simulink model "IEEE5BusSystemModel_std_UFLS"  (R2019b)
settings: Solver=ode4  StartTime=0.0  StopTime=300  MaxStep=1e-4  RelTol=1e-3
InitFcn:
  | startup_RTS
values from neighbouring files (symbols this model uses):
  C = b/(2*pi*60*Zn)    [startup_RTS.m]
  C0 = C/3    [startup_RTS.m]
  fn = 50    [startup_RTS.m]
  In = Sn/(sqrt(3)*Vn)    [startup_RTS.m]
  L = x*Zn/(2*pi*60)    [startup_RTS.m]
  L0 = 3*L    [startup_RTS.m]
  len = ceil(0.95*300000*T_prop)    [startup_RTS.m]
  PL1 = 300e6    (= 300000000)    [startup_RTS.m]
  PL2 = 300e6    (= 300000000)    [startup_RTS.m]
  PL3 = 300e6    (= 300000000)    [startup_RTS.m]
  QL1 = 30e6    (= 30000000)    [startup_RTS.m]
  QL2 = 30e6    (= 30000000)    [startup_RTS.m]
  QL3 = 30e6    (= 30000000)    [startup_RTS.m]
  R = r*Zn    [startup_RTS.m]
  R0 = 3*R    [startup_RTS.m]
  Sn = 1000e6    (= 1000000000)    [startup_RTS.m]
  t_cont = 100    [startup_RTS.m]
  Vn = 345e3    (= 345000)    [startup_RTS.m]
undefined symbols (not defined in the file or in its folder): D1, Delta
libraries: powerlib x42, powerlib_meascontrol x39, dspswit3 x10, dspstat3 x3, sps_avr x3, spsExcitationSystemModel x3
(part 1 of 7)
settings Model: Creator=Rodney Tan  LastModifiedBy=zuo
settings SolverCC: AutoInsertRateTranBlk=on
settings DataIOCC: ReturnWorkspaceOutputs=off
settings OptimizationCC: LifeSpan=inf
settings DebuggingCC: UnconnectedInputMsg=none  UnconnectedOutputMsg=none  UnconnectedLineMsg=none  SFUnexpectedBacktrackingDiag=warning  SFNoUnconditionalDefaultTransitionDiag=warning  SFExecutionAtInitializationDiag=none  ArithmeticOperatorsInVariantConditions=warning
settings SFSimCC: SimUseLocalCustomCode=off  CustomCodeUndefinedFunction=UseInterfaceOnly
settings RTWCC: RTWUseLocalCustomCode=off
settings CodeAppCC: StateflowObjectComments=on
settings GRTTargetCC: TargetLangStandard=C89/C90 (ANSI)  GeneratePreprocessorConditionals=Disable all
settings ConfigComp: CovMetricSettings=dw  CovHtmlReporting=on  CovSaveCumulativeToWorkspaceVar=on  CovSaveSingleToWorkspaceVar=on  CovExternalEMLEnable=off
settings SimscapeCC: SimscapeNormalizeSystem=off

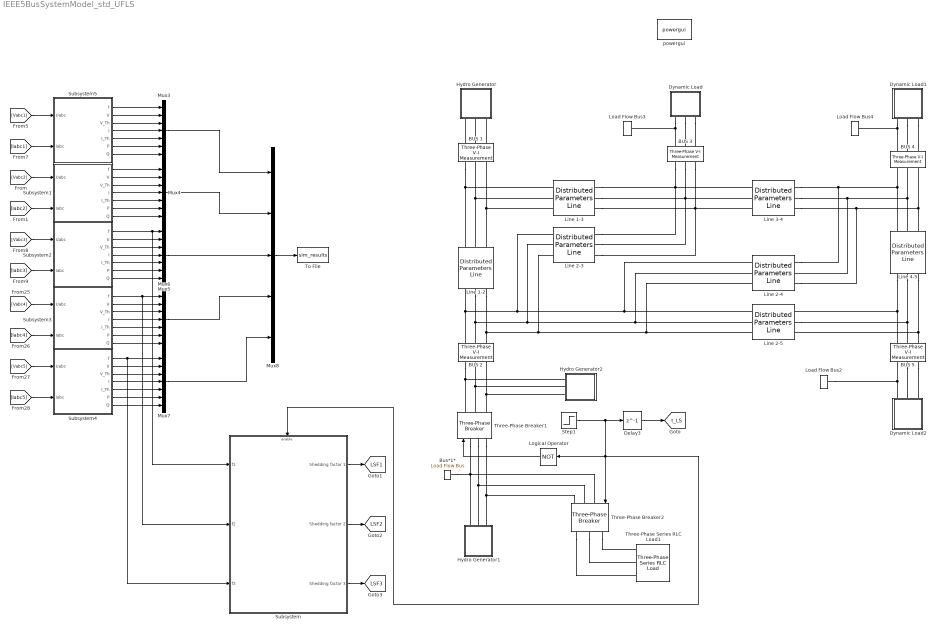
== system IEEE5BusSystemModel_std_UFLS ==
  BUS 1 : powerlib/Measurements/Three-Phase V-I Measurement  VoltageMeasurement=phase-to-ground  SetLabelV=on  LabelV=Vabc1  Vpu=off  VpuLL=off  CurrentMeasurement=yes  SetLabelI=on  LabelI=Iabc1  Ipu=off  Pbase=100e6  Vbase=500e3  OutputType=Complex  PhasorSimulation=off  PSBequivalent=0
      settings: SourceProductName=Simscape Electrical
  BUS 2 : powerlib/Measurements/Three-Phase V-I Measurement  VoltageMeasurement=phase-to-ground  SetLabelV=on  LabelV=Vabc2  Vpu=off  VpuLL=off  CurrentMeasurement=yes  SetLabelI=on  LabelI=Iabc2  Ipu=off  Pbase=100e6  Vbase=500e3  OutputType=Complex  PhasorSimulation=off  PSBequivalent=0
      settings: SourceProductName=Simscape Electrical
  BUS 3 : powerlib/Measurements/Three-Phase V-I Measurement  VoltageMeasurement=phase-to-ground  SetLabelV=on  LabelV=Vabc3  Vpu=off  VpuLL=off  CurrentMeasurement=yes  SetLabelI=on  LabelI=Iabc3  Ipu=off  Pbase=100e6  Vbase=500e3  OutputType=Complex  PhasorSimulation=off  PSBequivalent=0
      settings: SourceProductName=Simscape Electrical
  BUS 4 : powerlib/Measurements/Three-Phase V-I Measurement  VoltageMeasurement=phase-to-ground  SetLabelV=on  LabelV=Vabc4  Vpu=off  VpuLL=off  CurrentMeasurement=yes  SetLabelI=on  LabelI=Iabc4  Ipu=off  Pbase=100e6  Vbase=500e3  OutputType=Complex  PhasorSimulation=off  PSBequivalent=0
      settings: SourceProductName=Simscape Electrical
  BUS 5 : powerlib/Measurements/Three-Phase V-I Measurement  VoltageMeasurement=phase-to-ground  SetLabelV=on  LabelV=Vabc5  Vpu=off  VpuLL=off  CurrentMeasurement=yes  SetLabelI=on  LabelI=Iabc5  Ipu=off  Pbase=100e6  Vbase=500e3  OutputType=Complex  PhasorSimulation=off  PSBequivalent=0
      settings: SourceProductName=Simscape Electrical
  Bus*1* : powerlib/Measurements/Load Flow Bus  LConnTagsString=a  Phases=single  Connectors=on one side  ID=BUS_2_2  Vbase=345e3  Vref=1  Vangle=0  VLF=1.079  VLFb=1  VLFc=1  angleLF=22.73  angleLFb=0  angleLFc=0
      settings: SourceProductName=Simscape Electrical
  Delay3 : Delay  DelayLength=1  InitialCondition=0
  Dynamic Load : Subsystem
  Dynamic Load1 : Subsystem
  Dynamic Load2 : Subsystem
  Hydro Generator : Subsystem  mask{pTotal=1000, fNom=50, vNom=22}
      mask prompts: pTotal "Total generation (MWatt)"; fNom "Nominal frequency (Hz)"; vNom "Nominal L-L voltage (kV)"
      mask DialogControl ParameterGroupVar Prompt: HSG paramters
  Hydro Generator1 : Subsystem  mask{pTotal=1000, fNom=50, vNom=22}
      mask prompts: pTotal "Total generation (MWatt)"; fNom "Nominal frequency (Hz)"; vNom "Nominal L-L voltage (kV)"
      mask DialogControl ParameterGroupVar Prompt: HSG paramters
  Hydro Generator2 : Subsystem  mask{pTotal=1000, fNom=50, vNom=22}
      mask prompts: pTotal "Total generation (MWatt)"; fNom "Nominal frequency (Hz)"; vNom "Nominal L-L voltage (kV)"
      mask DialogControl ParameterGroupVar Prompt: HSG paramters
  Line 1-2 : powerlib/Elements/Distributed Parameters Line  Phases=3  Frequency=50  Resistance=[R(1) R0(1)]/len(1)  Inductance=[L(1) L0(1)]/len(1)  Capacitance=[C(1) C0(1)]/len(1)  Length=len(1)  x1=[-0.000175 -6.89085295701592e-11 283434.108559995 -241348.137066872;-0.00015 -2.16346671578411e-11 285320.892161224 -239114.627668055;-0.000125 2.56405297826555e-11 287190.075825844 -236866.368552673;-0.0001 7.29141450944975e-11 289041.544253801 -234603.498403938;-7.5e-05 1.20183262718414e-10 290875.183237801 -232326.156806341;-5e-05 1.67444966872572e-10 292690.879670354 -230034.484237038;-2.5e-05 2.14696342232437e-10 294488.521550753 -227728.622057188]  x2=[-0.000175 1.27432514229788e-09 287186.952133436 -239007.168100233;-0.00015 1.33160990762763e-09 289055.234274348 -236744.256496373;-0.000125 1.38881253298583e-09 290905.686126838 -234466.741391606;-0.0001 1.44592948984511e-09 292738.19354632 -232174.763273793;-7.5e-05 1.50295725496252e-09 294552.643495105 -229868.463522941;-5e-05 1.55989231059688e-09 296348.924049371 -227547.984402482;-2.5e-05 1.61673114472578e-09 298126.924406074 -225213.469050498]  x3=[-0.000175 -3.16049108701691e-11 2846.8299317029 -2460.69390485512;-0.00015 -3.08579762390022e-11 2866.06819220975 -2438.25927190657;-0.000125 -3.01091381425069e-11 2885.12966013012 -2415.6742356409;-0.0001 -2.93584427725443e-11 2904.01315966288 -2392.94018920953;-7.5e-05 -2.86059364355409e-11 2922.71752598482 -2370.05853495554;-5e-05 -2.78516655496321e-11 2941.24160532254 -2347.03068432714;-2.5e-05 -2.70956766417991e-11 2959.58425502355 -2323.85805779063]  x4=[-0.000175 3.74399132665437e-11 1776.05546983702 -1633.69511882766;-0.00015 3.68414015455268e-11 1788.83157054831 -1619.69575008179;-0.000125 3.6240617273324e-11 1801.49732770218 -1605.59647087261;-0.0001 3.56375975091392e-11 1814.05196001507 -1591.39815091007;-7.5e-05 3.5032379450072e-11 1826.49469305811 -1577.10166601343;-5e-05 3.44250004288231e-11 1838.82475930493 -1562.70789805721;-2.5e-05 3.38154979113915e-11 1851.04139817896 -1548.21773491684]  x5=0.000159154943091895  V1=ones(3,3)  V2=ones(3,3)  I1=ones(3,3)  I2=ones(3,3)  nHarmo=1  Measurements=None
      settings: SourceProductName=Simscape Electrical
  Line 1-3 : powerlib/Elements/Distributed Parameters Line  Phases=3  Frequency=50  Resistance=[R(2) R0(2)]/len(2)  Inductance=[L(2) L0(2)]/len(2)  Capacitance=[C(2) C0(2)]/len(2)  Length=len(2)  x1=[-0.0003 9.72648087730306e-10 277582.158753036 -250097.820068359;-0.000275 1.03025169047578e-09 279537.841922512 -247910.001458296;-0.00025 1.08779174244406e-09 281476.281881158 -245706.890591581;-0.000225 1.14526469429371e-09 283397.359056865 -243488.623366473;-0.0002 1.20266700082234e-09 285300.954948545 -241255.336616141;-0.000175 1.25999512118529e-09 287186.952133436 -239007.168100233;-0.00015 1.31724551911407e-09 289055.234274348 -236744.256496373;-0.000125 1.37441466313444e-09 290905.686126838 -234466.741391606;-0.0001 1.43149902678431e-09 292738.19354632 -232174.763273793;-7.5e-05 1.48849508883126e-09 294552.643495105 -229868.463522941;-5e-05 1.54539933348968e-09 296348.924049371 -227547.984402482;-2.5e-05 1.60220825063774e-09 298126.924406074 -225213.469050498]  x2=[-0.0003 1.7615419409433e-09 265030.630049931 -256880.545118797;-0.000275 1.80458215738261e-09 267039.971168693 -254791.095722945;-0.00025 1.84751105869411e-09 269032.840004163 -252685.929612136;-0.000225 1.89032599682095e-09 271009.113626804 -250565.176642931;-0.0002 1.93302433073608e-09 272968.670130749 -248428.967633363;-0.000175 1.97560342660514e-09 274911.388641323 -246277.434354866;-0.00015 2.01806065794892e-09 276837.149322498 -244110.709524149;-0.000125 2.0603934058054e-09 278745.833384283 -241928.926795004;-0.0001 2.10259905889129e-09 280637.323090054 -239732.220750067;-7.5e-05 2.1446750137631e-09 282511.501763818 -237520.726892514;-5e-05 2.18661867497775e-09 284368.253797405 -235294.581637705;-2.5e-05 2.22842745525262e-09 286207.464657603 -233053.922304763]  x3=[-0.0003 2.71909208464363e-11 572.658083588603 -630.300021251127;-0.000275 2.72692719095188e-11 577.590736411029 -625.782972903441;-0.00025 2.73459408754602e-11 582.487760716138 -621.227323314286;-0.000225 2.74209230149575e-11 587.348854432404 -616.633353497587;-0.0002 2.74942137027591e-11 592.173717704668 -612.001346831042;-0.000175 2.75658084179503e-11 596.962052912636 -607.33158903864;-0.00015 2.76357027442317e-11 601.713564689239 -602.624368173039;-0.000125 2.7703892370192e-11 606.427959938848 -597.879974597795;-0.0001 2.7770373089574e-11 611.104947855357 -593.098700969452;-7.5e-05 2.78351408015336e-11 615.744239940121 -588.280842219489;-5e-05 2.78981915108934e-11 620.345550019751 -583.426695536128;-2.5e-05 2.79595213283886e-11 624.908594263768 -578.536560346]  x4=[-0.0003 -2.32249180429763e-11 1364.78490116338 -1354.69627143181;-0.000275 -2.31577834751214e-11 1375.38246353659 -1343.93559538929;-0.00025 -2.30892204260988e-11 1385.89518584082 -1333.09201906874;-0.000225 -2.30192331252005e-11 1396.32241960183 -1322.16621135304;-0.0002 -2.29478258895727e-11 1406.66352161874 -1311.15884619745;-0.000175 -2.28750031239501e-11 1416.91785400366 -1300.07060258813;-0.00015 -2.2800769320384e-11 1427.08478422106 -1288.90216450015;-0.000125 -2.27251290579649e-11 1437.16368512681 -1277.6542208554;-0.0001 -2.26480870025407e-11 1447.15393500681 -1266.32746548002;-7.5e-05 -2.25696479064281e-11 1457.05491761539 -1254.92259706163;-5e-05 -2.24898166081201e-11 1466.86602221332 -1243.44031910624;-2.5e-05 -2.24085980319872e-11 1476.58664360543 -1231.88133989485]  x5=0.000290575841566274  V1=ones(3,3)  V2=ones(3,3)  I1=ones(3,3)  I2=ones(3,3)  nHarmo=1  Measurements=None
      settings: SourceProductName=Simscape Electrical
  Line 2-3 : powerlib/Elements/Distributed Parameters Line  Phases=3  Frequency=50  Resistance=[R(3) R0(3)]/len(3)  Inductance=[L(3) L0(3)]/len(3)  Capacitance=[C(3) C0(3)]/len(3)  Length=len(3)  x1=[-0.00025 -7.55210722613573e-10 277669.32737874 -247958.793830222;-0.000225 -7.06042606866762e-10 279608.208168973 -245770.356539619;-0.0002 -6.56830939086201e-10 281529.841407855 -243566.758975743;-0.000175 -6.07578754879368e-10 283434.108559994 -241348.137066872;-0.00015 -5.58289092352982e-10 285320.892161224 -239114.627668055;-0.000125 -5.08964991925604e-10 287190.075825844 -236866.368552673;-0.0001 -4.59609496140084e-10 289041.5442538 -234603.498403938;-7.5e-05 -4.10225649475888e-10 290875.1832378 -232326.156806341;-5e-05 -3.60816498161298e-10 292690.879670354 -230034.484237038;-2.5e-05 -3.11385089985503e-10 294488.521550752 -227728.622057188]  x2=[-0.00025 1.84751105869411e-09 269032.840004163 -252685.929612136;-0.000225 1.89032599682095e-09 271009.113626804 -250565.176642931;-0.0002 1.93302433073608e-09 272968.670130749 -248428.967633363;-0.000175 1.97560342660514e-09 274911.388641323 -246277.434354866;-0.00015 2.01806065794892e-09 276837.149322498 -244110.709524149;-0.000125 2.0603934058054e-09 278745.833384283 -241928.926795004;-0.0001 2.10259905889129e-09 280637.323090054 -239732.220750067;-7.5e-05 2.1446750137631e-09 282511.501763818 -237520.726892514;-5e-05 2.18661867497775e-09 284368.253797405 -235294.581637705;-2.5e-05 2.22842745525262e-09 286207.464657603 -233053.922304763]  x3=[-0.00025 2.75995009114326e-11 652.704108135299 -678.234675376389;-0.000225 2.79468601247303e-11 658.010768792704 -673.087474371481;-0.0002 2.82924954440539e-11 663.276840246383 -667.898754160629;-0.000175 2.8636385548989e-11 668.501997660243 -662.668834808537;-0.00015 2.8978509226774e-11 673.685918721962 -657.398038921264;-0.000125 2.9318845373609e-11 678.828283662869 -652.08669162633;-0.0001 2.96573729959572e-11 683.928775277674 -646.735120552653;-7.5e-05 2.99940712118403e-11 688.987078944027 -641.343655810347;-5e-05 3.03289192521264e-11 694.002882641933 -635.912629970351;-2.5e-05 3.0661896461811e-11 698.975876972991 -630.442378043924]  x4=[-0.00025 -2.89166148510431e-11 1397.97485671835 -1338.51479489178;-0.000225 -2.91605454608319e-11 1408.44430570704 -1327.49394730035;-0.0002 -2.94026773108183e-11 1418.82687521659 -1316.39121362919;-0.000175 -2.96429954651693e-11 1429.12192480121 -1305.20727874722;-0.00015 -2.98814850999289e-11 1439.32881941374 -1293.94283253223;-0.000125 -3.01181315039332e-11 1449.44692944484 -1282.5985698283;-0.0001 -3.03529200797173e-11 1459.47563076183 -1271.17519040301;-7.5e-05 -3.05858363444158e-11 1469.41430474717 -1259.67339890421;-5e-05 -3.08168659306565e-11 1479.26233833664 -1248.09390481657;-2.5e-05 -3.10459945874462e-11 1489.01912405713 -1236.43742241784]  x5=0.000225079079039277  V1=ones(3,3)  V2=ones(3,3)  I1=ones(3,3)  I2=ones(3,3)  nHarmo=1  Measurements=None
      settings: SourceProductName=Simscape Electrical
  Line 2-4 : powerlib/Elements/Distributed Parameters Line  Phases=3  Frequency=50  Resistance=[R(4) R0(4)]/len(4)  Inductance=[L(4) L0(4)]/len(4)  Capacitance=[C(4) C0(4)]/len(4)  Length=len(4)  x1=[-0.00025 -7.55210722613573e-10 277669.32737874 -247958.793830222;-0.000225 -7.06042606866762e-10 279608.208168973 -245770.356539619;-0.0002 -6.56830939086201e-10 281529.841407855 -243566.758975743;-0.000175 -6.07578754879368e-10 283434.108559994 -241348.137066872;-0.00015 -5.58289092352982e-10 285320.892161224 -239114.627668055;-0.000125 -5.08964991925604e-10 287190.075825844 -236866.368552673;-0.0001 -4.59609496140084e-10 289041.5442538 -234603.498403938;-7.5e-05 -4.10225649475888e-10 290875.1832378 -232326.156806341;-5e-05 -3.60816498161298e-10 292690.879670354 -230034.484237038;-2.5e-05 -3.11385089985503e-10 294488.521550752 -227728.622057188]  x2=[-0.00025 1.04438515929711e-09 268312.349842603 -253068.826139404;-0.000225 1.09016772438184e-09 270291.652916932 -250953.720015734;-0.0002 1.13588304278619e-09 272254.283128921 -248823.133884516;-0.000175 1.18152829457397e-09 274200.119414295 -246677.199170339;-0.00015 1.22710066413105e-09 276129.041744706 -244516.048244564;-0.000125 1.272597340339e-09 278040.931135137 -242339.814417159;-0.0001 1.31801551674853e-09 279935.669651247 -240148.631928479;-7.5e-05 1.36335239175258e-09 281813.140416638 -237942.63594098;-5e-05 1.40860516875915e-09 283673.227620069 -235721.962530887;-2.5e-05 1.45377105636378e-09 285515.816522601 -233486.748679795]  x3=[-0.00025 1.8608938054906e-11 620.73944245554 -651.189706585723;-0.000225 1.88719827024415e-11 625.834680289495 -646.294387025691;-0.0002 1.91338632371889e-11 630.891313692424 -641.359200983548;-0.000175 1.93945635051234e-11 635.909030747361 -636.384452884818;-0.00015 1.96540674250242e-11 640.887521937884 -631.370449595395;-0.000125 1.99123589894674e-11 645.826480167203 -626.31750040262;-0.0001 2.01694222658125e-11 650.725600777111 -621.225916996202;-7.5e-05 2.04252413971858e-11 655.584581566771 -616.096013448989;-5e-05 2.06798006034582e-11 660.403122811362 -610.928106197594;-2.5e-05 2.09330841822189e-11 665.180927280561 -605.722514022881]  x4=[-0.00025 -1.78719646829918e-11 1427.09295112561 -1366.9449250186;-0.000225 -1.80290498138173e-11 1437.78478964706 -1355.69450993648;-0.0002 -1.8185022827926e-11 1448.38793883011 -1344.36046923109;-0.000175 -1.83398741041675e-11 1458.90174462257 -1332.94350203946;-0.00015 -1.84935940905857e-11 1469.32555848339 -1321.44431261389;-0.000125 -1.86461733050078e-11 1479.65873742262 -1309.86361027857;-0.0001 -1.87976023356291e-11 1489.90064404111 -1298.20210938575;-7.5e-05 -1.89478718415938e-11 1500.05064656981 -1286.46052927175;-5e-05 -1.90969725535708e-11 1510.10811890877 -1274.63959421254;-2.5e-05 -1.9244895274326e-11 1520.07244066571 -1262.74003337907]  x5=0.000225079079039277  V1=ones(3,3)  V2=ones(3,3)  I1=ones(3,3)  I2=ones(3,3)  nHarmo=1  Measurements=None
      settings: SourceProductName=Simscape Electrical
  Line 2-5 : powerlib/Elements/Distributed Parameters Line  Phases=3  Frequency=50  Resistance=[R(5) R0(5)]/len(5)  Inductance=[L(5) L0(5)]/len(5)  Capacitance=[C(5) C0(5)]/len(5)  Length=len(5)  x1=[-0.000175 -6.07578754879368e-10 283434.108559994 -241348.137066872;-0.00015 -5.58289092352982e-10 285320.892161224 -239114.627668055;-0.000125 -5.08964991925604e-10 287190.075825844 -236866.368552673;-0.0001 -4.59609496140084e-10 289041.5442538 -234603.498403938;-7.5e-05 -4.10225649475888e-10 290875.1832378 -232326.156806341;-5e-05 -3.60816498161298e-10 292690.879670354 -230034.484237038;-2.5e-05 -3.11385089985503e-10 294488.521550752 -227728.622057188]  x2=[-0.000175 -1.8455816791541e-10 274204.431996219 -246369.649771894;-0.00015 -1.4365476424163e-10 276130.938727661 -244208.474456257;-0.000125 -1.02742499265318e-10 278040.412402109 -242032.23521159;-0.0001 -6.18238966476901e-11 279932.735234233 -239841.066278583;-7.5e-05 -2.09014804409006e-11 281807.790496646 -237635.102818854;-5e-05 2.00222250676572e-11 283665.462527109 -235414.480906623;-2.5e-05 6.09446955110597e-11 285505.636735659 -233179.337520308]  x3=[-0.000175 3.21776861319045e-11 522.866429808054 -510.097497337829;-0.00015 3.22539034337297e-11 526.856562179851 -505.975213824819;-0.000125 3.23281311628617e-11 530.814195557177 -501.821719377265;-0.0001 3.24003647405844e-11 534.739085814563 -497.637270202268;-7.5e-05 3.24705997111906e-11 538.63099084629 -493.422124416364;-5e-05 3.25388317422565e-11 542.489670581323 -489.176542029601;-2.5e-05 3.26050566249089e-11 546.31488699812 -484.900784929497]  x4=[-0.000175 -3.21081774868052e-11 1734.08510457111 -1566.21499511989;-0.00015 -3.20776836134101e-11 1746.33252307936 -1552.54734768471;-0.000125 -3.20452110373903e-11 1758.47221957162 -1538.78393181597;-0.0001 -3.20107617618073e-11 1770.50344521424 -1524.92559650599;-7.5e-05 -3.19743379116547e-11 1782.42545786453 -1510.97319660219;-5e-05 -3.19359417337271e-11 1794.23752211662 -1496.92759275429;-2.5e-05 -3.18955755964816e-11 1805.93890934672 -1482.78965136132]  x5=0.000159154943091895  V1=ones(3,3)  V2=ones(3,3)  I1=ones(3,3)  I2=ones(3,3)  nHarmo=1  Measurements=None
      settings: SourceProductName=Simscape Electrical
  Line 3-4 : powerlib/Elements/Distributed Parameters Line  Phases=3  Frequency=50  Resistance=[R(6) R0(6)]/len(6)  Inductance=[L(6) L0(6)]/len(6)  Capacitance=[C(6) C0(6)]/len(6)  Length=len(6)  x1=[-7.5e-05 2.14450359391277e-09 282511.501763818 -237520.726892514;-5e-05 2.18650438920275e-09 284368.253797405 -235294.581637705;-2.5e-05 2.22837031060265e-09 286207.464657603 -233053.922304763]  x2=[-7.5e-05 1.36335239175258e-09 281813.140416638 -237942.63594098;-5e-05 1.40860516875915e-09 283673.227620069 -235721.962530887;-2.5e-05 1.45377105636378e-09 285515.816522601 -233486.748679795]  x3=[-7.5e-05 -6.39975385908229e-11 1707.26151893148 -1486.29546105194;-5e-05 -6.42947165516981e-11 1718.8820864755 -1472.84094214289;-2.5e-05 -6.45879285116012e-11 1730.39662527578 -1459.29557146682]  x4=[-7.5e-05 5.80762461840834e-11 2107.15394566836 -1794.76808776156;-5e-05 5.87994680738186e-11 2121.18489524858 -1778.16333946726;-2.5e-05 5.95190629353929e-11 2135.08500015278 -1761.44890568229]  x5=6.49747334361397e-05  V1=ones(3,3)  V2=ones(3,3)  I1=ones(3,3)  I2=ones(3,3)  nHarmo=1  Measurements=None
      settings: SourceProductName=Simscape Electrical
  Line 4-5 : powerlib/Elements/Distributed Parameters Line  Phases=3  Frequency=50  Resistance=[R(7) R0(7)]/len(7)  Inductance=[L(7) L0(7)]/len(7)  Capacitance=[C(7) C0(7)]/len(7)  Length=len(7)  x1=[-0.0003 -4.02656590795237e-10 264320.598105925 -256944.934494444;-0.000275 -3.61902544883196e-10 266330.466826514 -254861.059625176;-0.00025 -3.21126175117472e-10 268323.907029381 -252761.463725248;-0.000225 -2.80329996776628e-10 270300.795749744 -250646.276307624;-0.0002 -2.39516526361111e-10 272261.011043794 -248515.627847028;-0.000175 -1.98688281438024e-10 274204.431996219 -246369.649771894;-0.00015 -1.57847780485833e-10 276130.938727661 -244208.474456257;-0.000125 -1.16997542739012e-10 278040.412402109 -242032.23521159;-0.0001 -7.6140088032647e-11 279932.735234233 -239841.066278583;-7.5e-05 -3.52779366470004e-11 281807.790496646 -237635.102818854;-5e-05 5.58639084795246e-12 283665.462527109 -235414.480906623;-2.5e-05 4.64503737480036e-11 285505.636735659 -233179.337520308]  x2=[-0.0003 9.5262958939744e-10 264304.214498806 -257252.077448191;-0.000275 9.98538171616254e-10 266316.495998673 -255168.321785816;-0.00025 1.04438515929711e-09 268312.349842603 -253068.826139404;-0.000225 1.09016772438184e-09 270291.652916932 -250953.720015734;-0.0002 1.13588304278619e-09 272254.283128921 -248823.133884516;-0.000175 1.18152829457397e-09 274200.119414295 -246677.199170339;-0.00015 1.22710066413105e-09 276129.041744706 -244516.048244564;-0.000125 1.272597340339e-09 278040.931135137 -242339.814417159;-0.0001 1.31801551674853e-09 279935.669651247 -240148.631928479;-7.5e-05 1.36335239175258e-09 281813.140416638 -237942.63594098;-5e-05 1.40860516875915e-09 283673.227620069 -235721.962530887;-2.5e-05 1.45377105636378e-09 285515.816522601 -233486.748679795]  x3=[-0.0003 -2.58292308145759e-12 930.888255854728 -1007.97476830205;-0.000275 -2.38221400636998e-12 938.776082330799 -1000.63256707165;-0.00025 -2.18135798510122e-12 946.606000676083 -993.228642111112;-0.000225 -1.98036740739683e-12 954.377527904332 -985.763450129404;-0.0002 -1.77925467130239e-12 962.09018463114 -978.237451614732;-0.000175 -1.57803218239878e-12 969.743495103511 -970.651110806135;-0.00015 -1.37671235303697e-12 977.336987229204 -963.004895664848;-0.000125 -1.17530760157233e-12 984.870192605857 -955.299277845438;-0.0001 -9.73830351598629e-13 992.342646549877 -947.53473266671;-7.5e-05 -7.72293031181692e-13 999.753888125107 -939.711739082384;-5e-05 -5.70708072092767e-13 1007.10346017126 -931.830779651553;-2.5e-05 -3.6908790904168e-13 1014.3909093321 -923.892340508919]  x4=[-0.0003 2.44800646108232e-12 953.120272984546 -1001.55052875308;-0.000275 2.36564734954155e-12 960.956958009434 -994.033917746149;-0.00025 2.28314231372906e-12 968.73436668264 -986.455990044854;-0.000225 2.2004964429441e-12 976.452019256962 -978.817213091471;-0.0002 2.11771483517327e-12 984.109439671238 -971.118058081744;-0.000175 2.03480259677608e-12 991.706155579704 -963.35899993582;-0.00015 1.95176484216995e-12 999.241698381142 -955.540517268954;-0.000125 1.86860669351472e-12 1006.71560324778 -947.663092361985;-0.0001 1.78533328039671e-12 1014.12740915395 -939.727211131587;-7.5e-05 1.7019497395123e-12 1021.47665890455 -931.733363100297;-5e-05 1.61846121435105e-12 1028.76289916325 -923.682041366314;-2.5e-05 1.53487285487847e-12 1035.98568048043 -915.573742573089]  x5=0.000290575841566274  V1=ones(3,3)  V2=ones(3,3)  I1=ones(3,3)  I2=ones(3,3)  nHarmo=1  Measurements=None
      settings: SourceProductName=Simscape Electrical
  Load Flow Bus2 : powerlib/Measurements/Load Flow Bus  LConnTagsString=a  Phases=single  Connectors=on one side  ID=BUS_5  Vbase=345e3  Vref=1  Vangle=0  VLF=1.068  VLFb=1  VLFc=1  angleLF=21.21  angleLFb=0  angleLFc=0
      settings: SourceProductName=Simscape Electrical
  Load Flow Bus3 : powerlib/Measurements/Load Flow Bus  LConnTagsString=a  Phases=single  Connectors=on one side  ID=BUS_3  Vbase=345e3  Vref=1  Vangle=0  VLF=1.07  VLFb=1  VLFc=1  angleLF=21.29  angleLFb=0  angleLFc=0
      settings: SourceProductName=Simscape Electrical
  Load Flow Bus4 : powerlib/Measurements/Load Flow Bus  LConnTagsString=a  Phases=single  Connectors=on one side  ID=BUS_4  Vbase=345e3  Vref=1  Vangle=0  VLF=1.069  VLFb=1  VLFc=1  angleLF=21.17  angleLFb=0  angleLFc=0
      settings: SourceProductName=Simscape Electrical
  Logical Operator : Logic  Operator=NOT  AllPortsSameDT=off  OutDataTypeStr=boolean
  Mux{3..7} (5 alike) : Mux  Inputs=7
  Mux8 : Mux  Inputs=5
  Step1 : Step  Time=t_cont  SampleTime=0
  Subsystem : Subsystem
  Subsystem1 : Subsystem
  Subsystem2 : Subsystem
  Subsystem3 : Subsystem
  Subsystem4 : Subsystem
  Subsystem5 : Subsystem
  Three-Phase Series RLC Load1 : powerlib/Elements/Three-Phase Series RLC Load  LConnTagsString=A|B|C  Configuration=Y (grounded)  NominalVoltage=(345000)*1.02511  Vabc=[1e3 1e3 1e3]  Vabcp=[1e3 1e3 1e3]  NominalFrequency=50  UnbalancedPower=off  ActivePower=300e6  InductivePower=30e6  CapacitivePower=0  Pabc=[10e3 9e3 11e3]  QLabc=[100 90 110]  QCabc=[100 90 110]  Pabcp=[10e3 9e3 11e3]  QLabcp=[100 90 110]  QCabcp=[100 90 110]  Measurements=None  LoadType=constant PQ
      settings: SourceProductName=Simscape Electrical
  Three-Phase Breaker1 : powerlib/Elements/Three-Phase Breaker  InitialState=closed  SwitchA=on  SwitchB=on  SwitchC=on  SwitchTimes=[]  External=on  BreakerResistance=0.01  SnubberResistance=1e9  SnubberCapacitance=inf  Measurements=None
      settings: SourceProductName=Simscape Electrical
  Three-Phase Breaker2 : powerlib/Elements/Three-Phase Breaker  InitialState=open  SwitchA=on  SwitchB=on  SwitchC=on  SwitchTimes=[]  External=on  BreakerResistance=0.01  SnubberResistance=1e9  SnubberCapacitance=inf  Measurements=None
      settings: SourceProductName=Simscape Electrical
  To File : ToFile  Filename=sim_results  MatrixName=sim1
  powergui : powerlib/powergui  Priority=1  SimulationMode=Discrete  SampleTime=25e-6  frequency=60  Iterations=50  frequencyindice=50  Pbase=1000e6  ErrMax=0.0001  UnitsV=kV  UnitsW=MW  buscounter=3  FunctionMessages=off  echomessages=off  EnableUseOfTLC=off  CurrentSourceSwitches=off  DisableSnubberDevices=off  DisableRonSwitches=off  DisableVfSwitches=off  DisplayEquations=off  AutomaticDiscreteSolvers=off  SolverType=Tustin/Backward Euler (TBE)  Interpol=off  ExternalGateDelay=off  methode=off  Ts=100  x0status=blocks  SPID=on  SwTol=0  HookPort=off  NonlinearTolerance=1e-4  nMaxIteration=100  ContinueOnMaxIteration=off  RestoreLinks=warning  ResistiveCurrentMeasurement=off  Frange=[0:2:500]  Ylog=off  Xlog=on  ShowGrid=off  save=off  variable=ZData  structure=0  ZoomFFT=off  StartTime=0.0  cycles=1  DisplayStyle=1  fundamental=60  FreqAxis=off  MaxFrequency=1000  frequencyindicesteady=1  RmsSteady=1  display=off
      settings: SourceProductName=Simscape Electrical
  tag scope: LSF1=global, LSF2=global, LSF3=global, t_LS=global
  wires:
  Logical Operator/1 -> Three-Phase Breaker1/1
  Step1/1 -> Logical Operator/1, Subsystem/Enable, Three-Phase Breaker2/1, Delay3/1
  [Vabc1] -> Subsystem5/1(Uabc)
  [Vabc3] -> Subsystem2/1(Uabc)
  [Iabc2] -> Subsystem1/2(Iabc)
  [Iabc3] -> Subsystem2/2(Iabc)
  [Iabc1] -> Subsystem5/2(Iabc)
  [Vabc2] -> Subsystem1/1(Uabc)
  [Vabc4] -> Subsystem3/1(Uabc)
  [Iabc5] -> Subsystem4/2(Iabc)
  [Iabc4] -> Subsystem3/2(Iabc)
  [Vabc5] -> Subsystem4/1(Uabc)
  Subsystem5/1(f) -> Mux3/1
  Subsystem5/2(V) -> Mux3/2
  Subsystem5/3(V_Th) -> Mux3/3
  Subsystem5/4(I) -> Mux3/4
  Subsystem5/5(I_Th) -> Mux3/5
  Subsystem5/6(P) -> Mux3/6
  Subsystem5/7(Q) -> Mux3/7
  Subsystem1/7(Q) -> Mux4/7
  Subsystem1/6(P) -> Mux4/6
  Subsystem1/5(I_Th) -> Mux4/5
  Subsystem1/4(I) -> Mux4/4
  Subsystem1/3(V_Th) -> Mux4/3
  Subsystem1/2(V) -> Mux4/2
  Subsystem1/1(f) -> Mux4/1
  Subsystem2/1(f) -> Subsystem/1(f1), Mux5/1
  Subsystem2/2(V) -> Mux5/2
  Subsystem2/3(V_Th) -> Mux5/3
  Subsystem2/4(I) -> Mux5/4
  Subsystem2/5(I_Th) -> Mux5/5
  Subsystem2/6(P) -> Mux5/6
  Subsystem2/7(Q) -> Mux5/7
  Subsystem3/7(Q) -> Mux6/7
  Subsystem3/6(P) -> Mux6/6
  Subsystem3/5(I_Th) -> Mux6/5
  Subsystem3/4(I) -> Mux6/4
  Subsystem3/3(V_Th) -> Mux6/3
  Subsystem3/2(V) -> Mux6/2
  Subsystem4/1(f) -> Subsystem/3(f3), Mux7/1
  Subsystem4/2(V) -> Mux7/2
  Subsystem4/3(V_Th) -> Mux7/3
  Subsystem4/4(I) -> Mux7/4
  Subsystem4/5(I_Th) -> Mux7/5
  Subsystem4/6(P) -> Mux7/6
  Subsystem4/7(Q) -> Mux7/7
  Mux8/1 -> To File/1
  Mux3/1 -> Mux8/1
  Mux4/1 -> Mux8/2
  Mux5/1 -> Mux8/3
  Mux6/1 -> Mux8/4
  Mux7/1 -> Mux8/5
  Delay3/1 -> [t_LS]
  Subsystem3/1(f) -> Subsystem/2(f2), Mux6/1
  Subsystem/1(Shedding factor 1) -> [LSF1]
  Subsystem/2(Shedding factor 2) -> [LSF2]
  Subsystem/3(Shedding factor 3) -> [LSF3]
  connections:
  BUS 5/RConn1 -- Line 4-5/LConn1 -- Line 2-5/RConn1
  Line 2-5/RConn2 -- Line 4-5/LConn2 -- BUS 5/RConn2
  BUS 5/RConn3 -- Line 4-5/LConn3 -- Line 2-5/RConn3
  BUS 1/LConn2 -- Hydro Generator/RConn2
  BUS 1/LConn3 -- Hydro Generator/RConn3
  BUS 1/LConn1 -- Hydro Generator/RConn1
  Dynamic Load1/LConn1 -- BUS 4/LConn1 -- Load Flow Bus4/LConn1
  Load Flow Bus2/LConn1 -- Dynamic Load2/LConn1 -- BUS 5/LConn1
  Dynamic Load/LConn1 -- Load Flow Bus3/LConn1 -- BUS 3/LConn1
  Dynamic Load/LConn2 -- BUS 3/LConn2
  Dynamic Load/LConn3 -- BUS 3/LConn3
  Dynamic Load1/LConn2 -- BUS 4/LConn2
  Dynamic Load1/LConn3 -- BUS 4/LConn3
  BUS 5/LConn2 -- Dynamic Load2/LConn2
  BUS 5/LConn3 -- Dynamic Load2/LConn3
  Three-Phase Breaker2/RConn1 -- Three-Phase Series RLC Load1/LConn1
  Three-Phase Breaker2/RConn2 -- Three-Phase Series RLC Load1/LConn2
  Three-Phase Breaker2/RConn3 -- Three-Phase Series RLC Load1/LConn3
  Hydro Generator1/RConn2 -- Three-Phase Breaker1/LConn2 -- Three-Phase Breaker2/LConn2
  BUS 1/RConn1 -- Line 1-3/LConn1 -- Line 1-2/RConn1
  BUS 1/RConn2 -- Line 1-3/LConn2 -- Line 1-2/RConn2
  Line 1-2/RConn3 -- Line 1-3/LConn3 -- BUS 1/RConn3
  BUS 2/RConn1 -- Line 2-3/LConn1 -- Line 2-5/LConn1 -- Line 2-4/LConn1 -- Line 1-2/LConn1
  BUS 2/RConn2 -- Line 2-3/LConn2 -- Line 2-5/LConn2 -- Line 2-4/LConn2 -- Line 1-2/LConn2
  BUS 2/RConn3 -- Line 2-3/LConn3 -- Line 2-5/LConn3 -- Line 2-4/LConn3 -- Line 1-2/LConn3
  BUS 3/RConn1 -- Line 3-4/LConn1 -- Line 1-3/RConn1 -- Line 2-3/RConn1
  BUS 3/RConn2 -- Line 3-4/LConn2 -- Line 2-3/RConn2 -- Line 1-3/RConn2
  BUS 3/RConn3 -- Line 3-4/LConn3 -- Line 2-3/RConn3 -- Line 1-3/RConn3
  Line 2-4/RConn1 -- Line 4-5/RConn1 -- BUS 4/RConn1 -- Line 3-4/RConn1
  BUS 4/RConn2 -- Line 4-5/RConn2 -- Line 3-4/RConn2 -- Line 2-4/RConn2
  Line 2-4/RConn3 -- Line 4-5/RConn3 -- BUS 4/RConn3 -- Line 3-4/RConn3
  Hydro Generator2/RConn3 -- Three-Phase Breaker1/RConn3 -- BUS 2/LConn3
  BUS 2/LConn1 -- Three-Phase Breaker1/RConn1 -- Hydro Generator2/RConn1
  Hydro Generator2/RConn2 -- BUS 2/LConn2 -- Three-Phase Breaker1/RConn2
  Hydro Generator1/RConn1 -- Three-Phase Breaker1/LConn1 -- Bus*1*/LConn1 -- Three-Phase Breaker2/LConn1
  Hydro Generator1/RConn3 -- Three-Phase Breaker1/LConn3 -- Three-Phase Breaker2/LConn3

== system IEEE5BusSystemModel_std_UFLS/Dynamic Load ==
  Bus_L8 : powerlib/Measurements/Three-Phase V-I Measurement  VoltageMeasurement=phase-to-ground  SetLabelV=off  LabelV=V_Bus_L8  Vpu=off  VpuLL=off  CurrentMeasurement=no  SetLabelI=on  LabelI=I_L8  Ipu=off  Pbase=100e6  Vbase=230e3  OutputType=Complex  PhasorSimulation=off  PSBequivalent=0
      settings: SourceProductName=Simscape Electrical
  Load 8 : Subsystem
  Mux : Mux  Inputs=2
  Mux1 : Mux  Inputs=2
  P0 : Constant  Value=PL1
  Product : Product
  Product1 : Product
  Q0 : Constant  Value=QL1
  Scope : Scope
  Switch : Switch  Threshold=1
  Terminator : Terminator
  Three-Phase Dynamic Load : powerlib/Elements/Three-Phase Dynamic Load  NominalVoltage=[345e3 50 ]  ActiveReactivePowers=[3e+08 3e+07]  PositiveSequence=[1.06983 21.2941]  ExternalControl=on  NpNq=[1.3 2]  TimeConstants="[0  0  0  0]"  MinimumVoltage=0.7  Tfilter=1e-4  LoadFlowParameters=[4,0,0,0,0]
      settings: SourceProductName=Simscape Electrical  SourceProductBaseCode=PS
  A : PMIOPort  Side=Left
  B : PMIOPort  Port=2  Side=Left
  C : PMIOPort  Port=3  Side=Left
  wires:
  Load 8/1(Load Power) -> Scope/1, Three-Phase Dynamic Load/1
  Three-Phase Dynamic Load/1 -> Terminator/1
  Bus_L8/1 -> Load 8/1(Vabc)
  P0/1 -> Product/1, Mux1/1
  [t_LS] -> Switch/2
  Mux1/1 -> Switch/3
  Mux/1 -> Switch/1
  Switch/1 -> Load 8/2("[P0,Q0]")
  Q0/1 -> Product1/2, Mux1/2
  [LSF1] -> Product1/1, Product/2
  Product/1 -> Mux/1
  Product1/1 -> Mux/2
  connections:
  Three-Phase Dynamic Load/LConn1 -- Bus_L8/RConn1
  C/RConn1 -- Bus_L8/LConn3
  B/RConn1 -- Bus_L8/LConn2
  A/RConn1 -- Bus_L8/LConn1
  Three-Phase Dynamic Load/LConn2 -- Bus_L8/RConn2
  Three-Phase Dynamic Load/LConn3 -- Bus_L8/RConn3

== system IEEE5BusSystemModel_std_UFLS/Dynamic Load1 ==
  Bus_L8 : powerlib/Measurements/Three-Phase V-I Measurement  VoltageMeasurement=phase-to-ground  SetLabelV=off  LabelV=V_Bus_L8  Vpu=off  VpuLL=off  CurrentMeasurement=no  SetLabelI=on  LabelI=I_L8  Ipu=off  Pbase=100e6  Vbase=230e3  OutputType=Complex  PhasorSimulation=off  PSBequivalent=0
      settings: SourceProductName=Simscape Electrical
  Load 8 : Subsystem
  Mux : Mux  Inputs=2
  Mux1 : Mux  Inputs=2
  P0 : Constant  Value=PL2
  Product : Product
  Product1 : Product
  Q0 : Constant  Value=QL2
  Scope : Scope
  Switch : Switch  Threshold=1
  Terminator : Terminator
  Three-Phase Dynamic Load : powerlib/Elements/Three-Phase Dynamic Load  NominalVoltage=[345e3 50 ]  ActiveReactivePowers=[3e+08 3e+07]  PositiveSequence=[1.06907 21.1742]  ExternalControl=on  NpNq=[1.3 2]  TimeConstants="[0  0  0  0]"  MinimumVoltage=0.7  Tfilter=1e-4  LoadFlowParameters=[4,0,0,0,0]
      settings: SourceProductName=Simscape Electrical  SourceProductBaseCode=PS
  A : PMIOPort  Side=Left
  B : PMIOPort  Port=2  Side=Left
  C : PMIOPort  Port=3  Side=Left
  wires:
  Bus_L8/1 -> Load 8/1(Vabc)
  Three-Phase Dynamic Load/1 -> Terminator/1
  Load 8/1(Load Power) -> Three-Phase Dynamic Load/1, Scope/1
  Switch/1 -> Load 8/2("[P0,Q0]")
  [t_LS] -> Switch/2
  P0/1 -> Product/1, Mux1/1
  [LSF2] -> Product1/1, Product/2
  Product1/1 -> Mux/2
  Q0/1 -> Product1/2, Mux1/2
  Product/1 -> Mux/1
  Mux1/1 -> Switch/3
  Mux/1 -> Switch/1
  connections:
  Three-Phase Dynamic Load/LConn3 -- Bus_L8/RConn3
  Three-Phase Dynamic Load/LConn2 -- Bus_L8/RConn2
  A/RConn1 -- Bus_L8/LConn1
  B/RConn1 -- Bus_L8/LConn2
  C/RConn1 -- Bus_L8/LConn3
  Three-Phase Dynamic Load/LConn1 -- Bus_L8/RConn1

== system IEEE5BusSystemModel_std_UFLS/Dynamic Load2 ==
  Bus_L8 : powerlib/Measurements/Three-Phase V-I Measurement  VoltageMeasurement=phase-to-ground  SetLabelV=off  LabelV=V_Bus_L8  Vpu=off  VpuLL=off  CurrentMeasurement=no  SetLabelI=on  LabelI=I_L8  Ipu=off  Pbase=100e6  Vbase=230e3  OutputType=Complex  PhasorSimulation=off  PSBequivalent=0
      settings: SourceProductName=Simscape Electrical
  Load 8 : Subsystem
  Mux : Mux  Inputs=2
  Mux1 : Mux  Inputs=2
  P0 : Constant  Value=PL3
  Product : Product
  Product1 : Product
  Q0 : Constant  Value=QL3
  Scope : Scope
  Switch : Switch  Threshold=1
  Terminator : Terminator
  Three-Phase Dynamic Load : powerlib/Elements/Three-Phase Dynamic Load  NominalVoltage=[345e3 50 ]  ActiveReactivePowers=[3e+08 3e+07]  PositiveSequence=[1.06848 21.2101]  ExternalControl=on  NpNq=[1.3 2]  TimeConstants="[0  0  0  0]"  MinimumVoltage=0.7  Tfilter=1e-4  LoadFlowParameters=[4,0,0,0,0]
      settings: SourceProductName=Simscape Electrical  SourceProductBaseCode=PS
  A : PMIOPort  Side=Left
  B : PMIOPort  Port=2  Side=Left
  C : PMIOPort  Port=3  Side=Left
  wires:
  Load 8/1(Load Power) -> Scope/1, Three-Phase Dynamic Load/1
  Three-Phase Dynamic Load/1 -> Terminator/1
  Bus_L8/1 -> Load 8/1(Vabc)
  Switch/1 -> Load 8/2("[P0,Q0]")
  [t_LS] -> Switch/2
  P0/1 -> Product/1, Mux1/1
  [LSF3] -> Product1/1, Product/2
  Product1/1 -> Mux/2
  Q0/1 -> Product1/2, Mux1/2
  Product/1 -> Mux/1
  Mux1/1 -> Switch/3
  Mux/1 -> Switch/1
  connections:
  Three-Phase Dynamic Load/LConn1 -- Bus_L8/RConn1
  C/RConn1 -- Bus_L8/LConn3
  B/RConn1 -- Bus_L8/LConn2
  A/RConn1 -- Bus_L8/LConn1
  Three-Phase Dynamic Load/LConn2 -- Bus_L8/RConn2
  Three-Phase Dynamic Load/LConn3 -- Bus_L8/RConn3

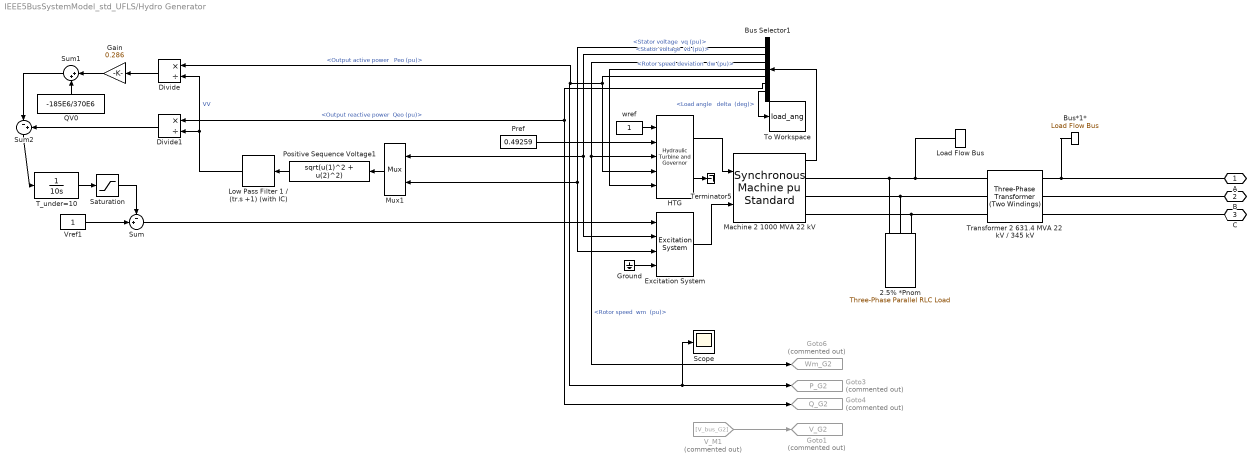
== system IEEE5BusSystemModel_std_UFLS/Hydro Generator ==
  2.5% *Pnom : powerlib/Elements/Three-Phase Parallel RLC Load  LConnTagsString=A|B|C  Configuration=Y (grounded)  NominalVoltage=vNom*1e3  Vabc=[1e3 1e3 1e3]  Vabcp=[1e3 1e3 1e3]  NominalFrequency=50  UnbalancedPower=off  ActivePower=pTotal*1e6*0.025  InductivePower=0  CapacitivePower=0  Pabc=[10e3 9e3 11e3]  QLabc=[100 90 110]  QCabc=[100 90 110]  Pabcp=[10e3 9e3 11e3]  QLabcp=[100 90 110]  QCabcp=[100 90 110]  Measurements=None  LoadType=constant Z
      settings: SourceProductName=Simscape Electrical
  Bus Selector1 : BusSelector  OutputSignals="dq0 components.Stator voltage  vq (pu),dq0 components.Stator voltage  vd (pu),Mechanical.Rotor speed  wm  (pu),Mechanical.Rotor speed deviation  dw (pu),Output active power   Peo (pu),Output reactive power  Qeo (pu),Load angle   delta  (deg)"
  Bus*1* : powerlib/Measurements/Load Flow Bus  LConnTagsString=a  Phases=single  Connectors=on one side  ID=BUS_1_2  Vbase=345e3  Vref=1  Vangle=0  VLF=1.083  VLFb=1  VLFc=1  angleLF=23.38  angleLFb=0  angleLFc=0
      settings: SourceProductName=Simscape Electrical
  Divide : Product  Inputs=*/
  Divide1 : Product  Inputs=*/
  Excitation System : sps_avr/Excitation System  tr=20e-3  reg=[ 200, 0.02 ]  exc=[ 1, 0 .19]  tgr=[ 0, 0 ]  damp=[ 0.0012, 1 ]  sat=[ 0, 0 ]  lim=[ 0, 7.32, 0 ]  v0=[1 1.2767]
      settings: SourceProductName=Simscape Electrical  SourceProductBaseCode=PS
  Gain : Gain  Gain=0.286
  Goto1 : Goto  Commented=on  GotoTag=V_G2  TagVisibility=global
  Goto3 : Goto  Commented=on  GotoTag=P_G2  TagVisibility=global
  Goto4 : Goto  Commented=on  GotoTag=Q_G2  TagVisibility=global
  Goto6 : Goto  Commented=on  GotoTag=Wm_G2  TagVisibility=global
  Ground : Ground
  HTG : powerlib/Machines/Hydraulic Turbine and Governor  sm="[ 10/3  0.07 ]"  gate="[  0.01  0.97518  -0.1  0.1 ]"  reg="[  0.05  1.163  0.105  0  0.01  ]"  hyd="[  0  2.67  ]"  dref=0  po=0.4938
      settings: SourceProductName=Simscape Electrical  SourceProductBaseCode=PS
  Load Flow Bus : powerlib/Measurements/Load Flow Bus  LConnTagsString=a  Phases=single  Connectors=on one side  ID=BUS_1_1  Vbase=22e3  Vref=1  Vangle=0  VLF=1  VLFb=1  VLFc=1  angleLF=0  angleLFb=0  angleLFc=0
      settings: SourceProductName=Simscape Electrical
  Low Pass Filter 1 / (tr.s +1) (with IC) : spsExcitationSystemModel/Discrete/Low Pass Filter 1 // (tr.s +1) (with IC)  FilterType=Lowpass  Tc=20e-3  Ts=25e-6  Initialize=on  Vac_Init=[0 0 50]  Vdc_Init=1  PlotResponse=off  param1=[1 500 0.1]
      settings: SourceProductName=Simscape Electrical  SourceProductBaseCode=PS
  Machine 2 1000 MVA 22 kV : powerlib/Machines/Synchronous Machine pu Standard  PresetModel=No  MechanicalLoad=Mechanical power Pm  ShowDetailedParameters=on  RotorType=Round  Units=per unit standard parameters  MeasurementBus=off  NominalParameters=[pTotal*1e+006 vNom*1e3 fNom]  Reactances1=[ 1.693 0.4 0.2 1.618 0.967 0.2 0.035 ]  Reactances2=[1.699 0.174 0.109 0.838 0.185 0.069]  dAxisTimeConstants=Open-circuit  qAxisTimeConstants=Open-circuit  TimeConstants1=[]  TimeConstants2=[6.56 0.03 1.5 0.04]  TimeConstants3=[]  TimeConstants4=[]  TimeConstants5=[ 9.2, 0.01, 0.01 ]  TimeConstants6=[]  TimeConstants7=[0.024 0.006 0.006]  TimeConstants8=[1 2 3 1]  StatorResistance=0.005  Mechanical=[5.28 0.02558 2]  PolePairs=2  InitialConditions=[0 -50.5494 0.493028 0.493028 0.493028 2.42806 -117.572 122.428 1.27674]  SetSaturation=off  Saturation=[0.6404,0.7127,0.8441,0.9214,0.9956,1.082,1.19,1.316,1.457;0.7,0.7698,0.8872,0.9466,0.9969,1.046,1.1,1.151,1.201]  LoadFlowParameters=[1 524200000 21604 0]  TsPowergui=0  TsBlock=-1  IterativeModel=Trapezoidal non iterative  IterativeDiscreteModel=Trapezoidal non iterative  BusType=swing  Pref=5.242e+008  Qref=0  Qmin=-Inf  Qmax=Inf  PLF=0  QLF=0
      settings: AttributesFormatString=\n\n  SourceProductName=Simscape Electrical
  Mux1 : Mux  Inputs=2
  Positive Sequence Voltage1 : Fcn  Expr=sqrt(u(1)^2 + u(2)^2)
  Pref : Constant  Value=0.49259
  QV0 : Constant  Value=-185E6/370E6
  Saturation : Saturate  UpperLimit=0  LowerLimit=-10
  Scope : Scope
  Sum : Sum  Inputs=-+|
  Sum1 : Sum  Inputs=|++
  Sum2 : Sum  Inputs=|-+
  T_under=10 : TransferFcn  Denominator=[10 0 ]
  Terminator5 : Terminator
  To Workspace : ToWorkspace  VariableName=load_ang  SampleTime=-1
      settings: Decimation=800  Save2DSignal=2-D array (concatenate along first dimension)
  Transformer 2 631.4 MVA 22 kV / 345 kV : powerlib/Elements/Three-Phase Transformer (Two Windings)  Winding1Connection=Delta (D1)  Winding2Connection=Yg  CoreType=Three single-phase transformers  SetSaturation=off  Hysteresis=off  DataFile='hysteresis'  SetInitialFlux=off  Measurements=None  UNITS=pu  NominalPower=[ pTotal*1e+6 fNom ]  Winding1="[vNom*1e3   0.0001     0.025*pTotal/100/2]"  Winding2="[ 1.07*345e3  0.0001     0.025*pTotal/100/2 ]"  Rm=500  Lm=500  L0=0.5  Saturation="[ 0,0  ;  0.005,1.2  ;  1.0,1.4 ]"  InitialFluxes=[ 0.8 , -0.8 , 0.7 ]  BreakLoop=off  DiscreteSolver=Trapezoidal iterative  DataType=off  TransfoNumber=0
      settings: SourceProductName=Simscape Electrical
  V_M1 : From  Commented=on  GotoTag=V_bus_G2
  Vref1 : Constant
  wref : Constant
  A : PMIOPort  Side=Right
  B : PMIOPort  Port=2  Side=Right
  C : PMIOPort  Port=3  Side=Right
  wires:
  Ground/1 -> Excitation System/4
  HTG/2 -> Terminator5/1
  Sum/1 -> Excitation System/1
  wref/1 -> HTG/1
  Excitation System/1 -> Machine 2 1000 MVA 22 kV/2
  HTG/1 -> Machine 2 1000 MVA 22 kV/1
  Machine 2 1000 MVA 22 kV/1 -> Bus Selector1/1
  Bus Selector1/3 -> HTG/3, Goto6/1  "<Rotor speed  wm  (pu)>"
  Bus Selector1/4 -> HTG/5  "<Rotor speed deviation  dw (pu)>"
  V_M1/1 -> Goto1/1
  Pref/1 -> HTG/2
  Bus Selector1/7 -> To Workspace/1  "<Load angle   delta  (deg)>"
  Saturation/1 -> Sum/1
  Gain/1 -> Sum1/1
  Sum1/1 -> Sum2/1
  Positive Sequence Voltage1/1 -> Low Pass Filter 1 / (tr.s +1) (with IC)/1
  Vref1/1 -> Sum/2
  Bus Selector1/5 -> HTG/4, Divide/1, Scope/1, Goto3/1  "<Output active power   Peo (pu)>"
  Divide/1 -> Gain/1
  Low Pass Filter 1 / (tr.s +1) (with IC)/1 -> Divide1/2, Divide/2  "VV"
  QV0/1 -> Sum1/2
  Sum2/1 -> T_under=10/1
  T_under=10/1 -> Saturation/1
  Mux1/1 -> Positive Sequence Voltage1/1
  Divide1/1 -> Sum2/2
  Bus Selector1/6 -> Divide1/1, Goto4/1  "<Output reactive power  Qeo (pu)>"
  Bus Selector1/1 -> Mux1/2, Excitation System/3  "<Stator voltage  vq (pu)>"
  Bus Selector1/2 -> Mux1/1, Excitation System/2  "<Stator voltage  vd (pu)>"
  connections:
  A/RConn1 -- Bus*1*/LConn1 -- Transformer 2 631.4 MVA 22 kV / 345 kV/RConn1
  B/RConn1 -- Transformer 2 631.4 MVA 22 kV / 345 kV/RConn2
  C/RConn1 -- Transformer 2 631.4 MVA 22 kV / 345 kV/RConn3
  2.5% *Pnom/LConn3 -- Transformer 2 631.4 MVA 22 kV / 345 kV/LConn3 -- Machine 2 1000 MVA 22 kV/RConn3
  2.5% *Pnom/LConn1 -- Load Flow Bus/LConn1 -- Transformer 2 631.4 MVA 22 kV / 345 kV/LConn1 -- Machine 2 1000 MVA 22 kV/RConn1
  Transformer 2 631.4 MVA 22 kV / 345 kV/LConn2 -- 2.5% *Pnom/LConn2 -- Machine 2 1000 MVA 22 kV/RConn2

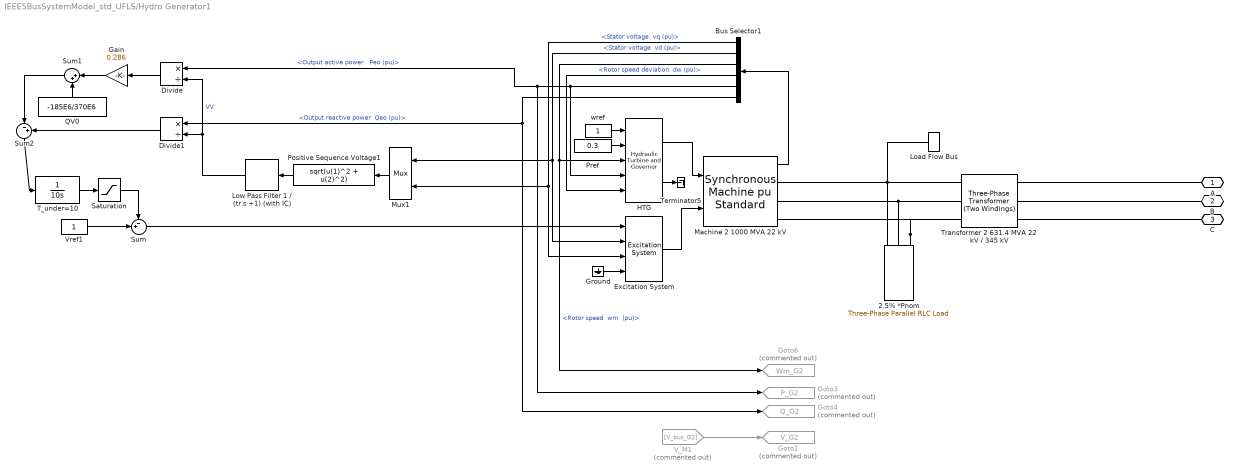
== system IEEE5BusSystemModel_std_UFLS/Hydro Generator1 ==
  2.5% *Pnom : powerlib/Elements/Three-Phase Parallel RLC Load  LConnTagsString=A|B|C  Configuration=Y (grounded)  NominalVoltage=vNom*1e3  Vabc=[1e3 1e3 1e3]  Vabcp=[1e3 1e3 1e3]  NominalFrequency=50  UnbalancedPower=off  ActivePower=pTotal*1e6*0.025  InductivePower=0  CapacitivePower=0  Pabc=[10e3 9e3 11e3]  QLabc=[100 90 110]  QCabc=[100 90 110]  Pabcp=[10e3 9e3 11e3]  QLabcp=[100 90 110]  QCabcp=[100 90 110]  Measurements=None  LoadType=constant Z
      settings: SourceProductName=Simscape Electrical
  Bus Selector1 : BusSelector  OutputSignals="dq0 components.Stator voltage  vq (pu),dq0 components.Stator voltage  vd (pu),Mechanical.Rotor speed  wm  (pu),Mechanical.Rotor speed deviation  dw (pu),Output active power   Peo (pu),Output reactive power  Qeo (pu)"
  Divide : Product  Inputs=*/
  Divide1 : Product  Inputs=*/
  Excitation System : sps_avr/Excitation System  tr=20e-3  reg=[ 200, 0.02 ]  exc=[ 1, 0 .19]  tgr=[ 0, 0 ]  damp=[ 0.0012, 1 ]  sat=[ 0, 0 ]  lim=[ 0, 7.32, 0 ]  v0=[1 1.0876]
      settings: SourceProductName=Simscape Electrical  SourceProductBaseCode=PS
  Gain : Gain  Gain=0.286
  Goto1 : Goto  Commented=on  GotoTag=V_G2  TagVisibility=global
  Goto3 : Goto  Commented=on  GotoTag=P_G2  TagVisibility=global
  Goto4 : Goto  Commented=on  GotoTag=Q_G2  TagVisibility=global
  Goto6 : Goto  Commented=on  GotoTag=Wm_G2  TagVisibility=global
  Ground : Ground
  HTG : powerlib/Machines/Hydraulic Turbine and Governor  sm="[ 10/3  0.07 ]"  gate="[  0.01  0.97518  -0.1  0.1 ]"  reg="[  0.05  1.163  0.105  0  0.01  ]"  hyd="[  0  2.67  ]"  dref=0  po=0.30045
      settings: SourceProductName=Simscape Electrical  SourceProductBaseCode=PS
  Load Flow Bus : powerlib/Measurements/Load Flow Bus  LConnTagsString=a  Phases=single  Connectors=on one side  ID=BUS_2_1  Vbase=22e3  Vref=1  Vangle=0  VLF=1  VLFb=1  VLFc=1  angleLF=-3.37  angleLFb=0  angleLFc=0
      settings: SourceProductName=Simscape Electrical
  Low Pass Filter 1 / (tr.s +1) (with IC) : spsExcitationSystemModel/Discrete/Low Pass Filter 1 // (tr.s +1) (with IC)  FilterType=Lowpass  Tc=20e-3  Ts=25e-6  Initialize=on  Vac_Init=[0 0 50]  Vdc_Init=1  PlotResponse=off  param1=[1 500 0.1]
      settings: SourceProductName=Simscape Electrical  SourceProductBaseCode=PS
  Machine 2 1000 MVA 22 kV : powerlib/Machines/Synchronous Machine pu Standard  PresetModel=No  MechanicalLoad=Mechanical power Pm  ShowDetailedParameters=on  RotorType=Round  Units=per unit standard parameters  MeasurementBus=off  NominalParameters=[pTotal*1e+006 vNom*1e3 fNom]  Reactances1=[ 1.693 0.4 0.2 1.618 0.967 0.2 0.035 ]  Reactances2=[1.699 0.174 0.109 0.838 0.185 0.069]  dAxisTimeConstants=Open-circuit  qAxisTimeConstants=Open-circuit  TimeConstants1=[]  TimeConstants2=[6.56 0.03 1.5 0.04]  TimeConstants3=[]  TimeConstants4=[]  TimeConstants5=[ 9.2, 0.01, 0.01 ]  TimeConstants6=[]  TimeConstants7=[0.024 0.006 0.006]  TimeConstants8=[1 2 3 1]  StatorResistance=0.005  Mechanical=[5.28 0.02558 2]  PolePairs=2  InitialConditions=[0 -66.6282 0.300914 0.300914 0.300914 1.09582 -118.904 121.096 1.08755]  SetSaturation=off  Saturation=[0.6404,0.7127,0.8441,0.9214,0.9956,1.082,1.19,1.316,1.457;0.7,0.7698,0.8872,0.9466,0.9969,1.046,1.1,1.151,1.201]  LoadFlowParameters=[1 524200000 21604 0]  TsPowergui=0  TsBlock=-1  IterativeModel=Trapezoidal non iterative  IterativeDiscreteModel=Trapezoidal non iterative  BusType=PV  Pref=300e6  Qref=0  Qmin=-100e6  Qmax=100e6  PLF=0  QLF=0
      settings: AttributesFormatString=\n\n  SourceProductName=Simscape Electrical
  Mux1 : Mux  Inputs=2
  Positive Sequence Voltage1 : Fcn  Expr=sqrt(u(1)^2 + u(2)^2)
  Pref : Constant  Value=0.3
  QV0 : Constant  Value=-185E6/370E6
  Saturation : Saturate  UpperLimit=0  LowerLimit=-10
  Sum : Sum  Inputs=-+|
  Sum1 : Sum  Inputs=|++
  Sum2 : Sum  Inputs=|-+
  T_under=10 : TransferFcn  Denominator=[10 0 ]
  Terminator5 : Terminator
  Transformer 2 631.4 MVA 22 kV / 345 kV : powerlib/Elements/Three-Phase Transformer (Two Windings)  Winding1Connection=Delta (D1)  Winding2Connection=Yg  CoreType=Three single-phase transformers  SetSaturation=off  Hysteresis=off  DataFile='hysteresis'  SetInitialFlux=off  Measurements=None  UNITS=pu  NominalPower=[ pTotal*1e+6 fNom ]  Winding1="[vNom*1e3   0.0     0.025*pTotal/100/2]"  Winding2="[ 1.07*345e3  0.0     0.025*pTotal/100/2 ]"  Rm=500  Lm=500  L0=0.5  Saturation="[ 0,0  ;  0.005,1.2  ;  1.0,1.4 ]"  InitialFluxes=[ 0.8 , -0.8 , 0.7 ]  BreakLoop=off  DiscreteSolver=Trapezoidal iterative  DataType=off  TransfoNumber=0
      settings: SourceProductName=Simscape Electrical
  V_M1 : From  Commented=on  GotoTag=V_bus_G2
  Vref1 : Constant
  wref : Constant
  A : PMIOPort  Side=Right
  B : PMIOPort  Port=2  Side=Right
  C : PMIOPort  Port=3  Side=Right
  wires:
  V_M1/1 -> Goto1/1
  Bus Selector1/4 -> HTG/5  "<Rotor speed deviation  dw (pu)>"
  Bus Selector1/3 -> Goto6/1, HTG/3  "<Rotor speed  wm  (pu)>"
  Machine 2 1000 MVA 22 kV/1 -> Bus Selector1/1
  HTG/1 -> Machine 2 1000 MVA 22 kV/1
  Excitation System/1 -> Machine 2 1000 MVA 22 kV/2
  wref/1 -> HTG/1
  Pref/1 -> HTG/2
  Sum/1 -> Excitation System/1
  HTG/2 -> Terminator5/1
  Ground/1 -> Excitation System/4
  Saturation/1 -> Sum/1
  Gain/1 -> Sum1/1
  Sum1/1 -> Sum2/1
  Positive Sequence Voltage1/1 -> Low Pass Filter 1 / (tr.s +1) (with IC)/1
  Vref1/1 -> Sum/2
  Bus Selector1/5 -> Divide/1, Goto3/1, HTG/4  "<Output active power   Peo (pu)>"
  Divide/1 -> Gain/1
  Low Pass Filter 1 / (tr.s +1) (with IC)/1 -> Divide1/2, Divide/2  "VV"
  QV0/1 -> Sum1/2
  Sum2/1 -> T_under=10/1
  T_under=10/1 -> Saturation/1
  Mux1/1 -> Positive Sequence Voltage1/1
  Divide1/1 -> Sum2/2
  Bus Selector1/6 -> Goto4/1, Divide1/1  "<Output reactive power  Qeo (pu)>"
  Bus Selector1/1 -> Excitation System/3, Mux1/2  "<Stator voltage  vq (pu)>"
  Bus Selector1/2 -> Excitation System/2, Mux1/1  "<Stator voltage  vd (pu)>"
  connections:
  2.5% *Pnom/LConn3 -- Transformer 2 631.4 MVA 22 kV / 345 kV/LConn3 -- Machine 2 1000 MVA 22 kV/RConn3
  B/RConn1 -- Transformer 2 631.4 MVA 22 kV / 345 kV/RConn2
  A/RConn1 -- Transformer 2 631.4 MVA 22 kV / 345 kV/RConn1
  Machine 2 1000 MVA 22 kV/RConn2 -- Transformer 2 631.4 MVA 22 kV / 345 kV/LConn2 -- 2.5% *Pnom/LConn2
  2.5% *Pnom/LConn1 -- Machine 2 1000 MVA 22 kV/RConn1 -- Transformer 2 631.4 MVA 22 kV / 345 kV/LConn1 -- Load Flow Bus/LConn1
  C/RConn1 -- Transformer 2 631.4 MVA 22 kV / 345 kV/RConn3
